simulink subsystem "consigna_torque_y_compensaciones"  (R2023b)
settings: Solver=VariableStepAuto  StartTime=0.0  StopTime=10.0  RelTol=1e-3
values from neighbouring files (symbols this model uses):
  b_eq = 2.1944e-5    (= 2.1944e-05)    [diagrama_polos_y_ceros_LTI.m]    (also in main.m = 2.19444444444e-05; parametros.m = 2.19444444444e-05)
  k_l = 0.25    [main.m]    (also in parametros.m)
  L_d = 6.6    [main.m]    (also in parametros.m = 0.0066)
  L_q = 5.8e-3    (= 0.0058)    [diagrama_polos_y_ceros_LTI.m]    (also in main.m = 5.8; parametros.m; variacion_de_parametros.m)
  lambda_m = 0.016    [main.m]    (also in parametros.m)
  P_p = 3    [diagrama_polos_y_ceros_LTI.m]    (also in main.m; parametros.m; variacion_de_parametros.m)
  r = 120.0    (= 120)    [diagrama_polos_y_ceros_LTI.m]    (also in main.m; parametros.m)
settings Model: Creator=nicol  LastModifiedBy=nicol

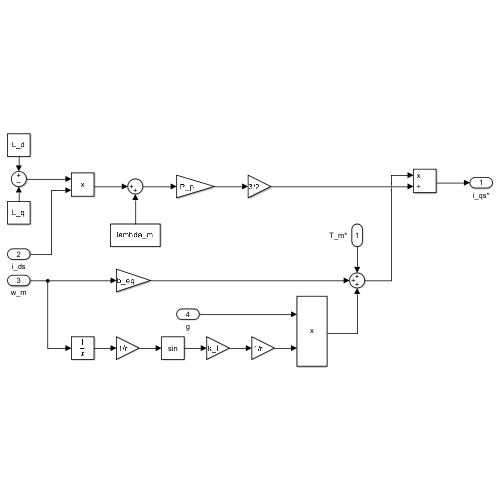
[thumbnail: Simulink's stored preview of the top-level diagram]
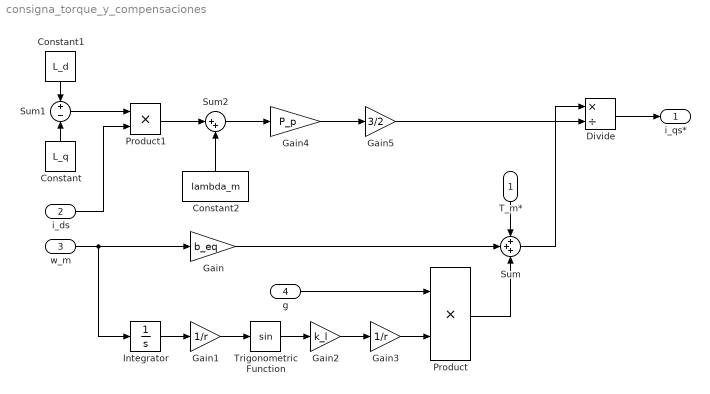
== system consigna_torque_y_compensaciones ==
  T_m* : Inport
  i_ds : Inport  Port=2
  w_m : Inport  Port=3
  g : Inport  Port=4
  Constant : Constant  Value=L_q
  Constant1 : Constant  Value=L_d
  Constant2 : Constant  Value=lambda_m
  Divide : Product  Inputs=*/
  Gain : Gain  Gain=b_eq
  Gain1 : Gain  Gain=1/r
  Gain2 : Gain  Gain=k_l
  Gain3 : Gain  Gain=1/r
  Gain4 : Gain  Gain=P_p
  Gain5 : Gain  Gain=3/2
  Integrator : Integrator
  Product : Product
  Product1 : Product
  Sum : Sum  Inputs=+++
  Sum1 : Sum  Inputs=+|-
  Sum2 : Sum  Inputs=|++
  Trigonometric Function : Trigonometry
  i_qs* : Outport
  wires:
  w_m/1 -> Gain/1, Integrator/1
  g/1 -> Product/1
  Gain3/1 -> Product/2
  Gain2/1 -> Gain3/1
  Trigonometric Function/1 -> Gain2/1
  Gain1/1 -> Trigonometric Function/1
  Integrator/1 -> Gain1/1
  Gain/1 -> Sum/2
  Product/1 -> Sum/3
  T_m*/1 -> Sum/1
  Sum/1 -> Divide/1
  Constant1/1 -> Sum1/1
  Constant/1 -> Sum1/2
  Sum1/1 -> Product1/1
  i_ds/1 -> Product1/2
  Product1/1 -> Sum2/1
  Constant2/1 -> Sum2/2
  Gain4/1 -> Gain5/1
  Sum2/1 -> Gain4/1
  Gain5/1 -> Divide/2
  Divide/1 -> i_qs*/1
